simulink model "HDVPSG_DelayComp_NewRef_RealDrop_case1"  (R2019b)
settings: Solver=FixedStepDiscrete  StartTime=0.0  StopTime=28  FixedStep=UT.Ts_Veh  RelTol=1e-3
PostLoadFcn:
  | if any(exist('dsrtsu_mdlpostloadfcn', 'file') ~= 0), dsrtsu_mdlpostloadfcn('Execute', bdroot); end
InitFcn:
  | , if any(exist('dsmpb_private', 'file') ~= 0), dsmpb_private('dsmpb_mdlclblib', 'Init', bdroot); end,
values from neighbouring files (symbols this model uses):
  BETA_HDV_Leader = 50    [HDVPSG_DelayComp_NewRef_RealDrop_script_case1.m]
  BETA_PSG_Follower = 150    [HDVPSG_DelayComp_NewRef_RealDrop_script_case1.m]
  CtrlZone_Length = 250    [HDVPSG_DelayComp_NewRef_RealDrop_script_case1.m]
  DELTA_D_MIN = 5    [HDVPSG_DelayComp_NewRef_RealDrop_script_case1.m]
  DELTA_DR_MG_TCC = 15    [HDVPSG_DelayComp_NewRef_RealDrop_script_case1.m]
  HDV_AMAX = 1.3    [HDVPSG_DelayComp_NewRef_RealDrop_script_case1.m]
  HDV_AMIN = -2.5    [HDVPSG_DelayComp_NewRef_RealDrop_script_case1.m]
  HDV_first_v0 = 13    [HDVPSG_DelayComp_NewRef_RealDrop_script_case1.m]
  HDV_HighMu_D = 9    [HDVPSG_DelayComp_NewRef_RealDrop_script_case1.m]
  HDV_HighMu_I = 27    [HDVPSG_DelayComp_NewRef_RealDrop_script_case1.m]
  HDV_HighMu_P = 27    [HDVPSG_DelayComp_NewRef_RealDrop_script_case1.m]
  HDV_HighMu_TRFC = 0.7    [HDVPSG_DelayComp_NewRef_RealDrop_script_case1.m]
  HDV_last_v0 = 13    [HDVPSG_DelayComp_NewRef_RealDrop_script_case1.m]
  HDV_LowMu_D = 6    [HDVPSG_DelayComp_NewRef_RealDrop_script_case1.m]
  HDV_LowMu_I = 8    [HDVPSG_DelayComp_NewRef_RealDrop_script_case1.m]
  HDV_LowMu_P = 12    [HDVPSG_DelayComp_NewRef_RealDrop_script_case1.m]
  HDV_LowMu_TRFC = 0.6    [HDVPSG_DelayComp_NewRef_RealDrop_script_case1.m]
  Np_MPC = 20    [HDVPSG_DelayComp_NewRef_RealDrop_script_case1.m]
  PSG_AMAX = 3.2    [HDVPSG_DelayComp_NewRef_RealDrop_script_case1.m]
  PSG_AMIN = -6    [HDVPSG_DelayComp_NewRef_RealDrop_script_case1.m]
  PSG_end_v0 = 13    [HDVPSG_DelayComp_NewRef_RealDrop_script_case1.m]
  PSG_first_v0 = 13    [HDVPSG_DelayComp_NewRef_RealDrop_script_case1.m]
  PSG_HighMu_D = 15    [HDVPSG_DelayComp_NewRef_RealDrop_script_case1.m]
  PSG_HighMu_I = 125    [HDVPSG_DelayComp_NewRef_RealDrop_script_case1.m]
  PSG_HighMu_P = 75    [HDVPSG_DelayComp_NewRef_RealDrop_script_case1.m]
  PSG_HighMu_TRFC = 0.8    [HDVPSG_DelayComp_NewRef_RealDrop_script_case1.m]
  PSG_LowMu_D = 12    [HDVPSG_DelayComp_NewRef_RealDrop_script_case1.m]
  PSG_LowMu_I = 64    [HDVPSG_DelayComp_NewRef_RealDrop_script_case1.m]
  PSG_LowMu_P = 48    [HDVPSG_DelayComp_NewRef_RealDrop_script_case1.m]
  PSG_LowMu_TRFC = 0.7    [HDVPSG_DelayComp_NewRef_RealDrop_script_case1.m]
  PSG_middle_v0 = 13    [HDVPSG_DelayComp_NewRef_RealDrop_script_case1.m]
  Q_Leader = 1    [HDVPSG_DelayComp_NewRef_RealDrop_script_case1.m]
  Qd_dot_PSG_Follower = 2    [HDVPSG_DelayComp_NewRef_RealDrop_script_case1.m]
  Qd_PSG_Follower = 10    [HDVPSG_DelayComp_NewRef_RealDrop_script_case1.m]
  R_Leader = 20    [HDVPSG_DelayComp_NewRef_RealDrop_script_case1.m]
  R_PSG_Follower = 1    [HDVPSG_DelayComp_NewRef_RealDrop_script_case1.m]
  Recved_40_1 = Recved_Flag_Combined(47740,:)    [HDVPSG_DelayComp_NewRef_RealDrop_script_case1.m]
  Recved_40_2 = Recved_Flag_Combined(47780,:)    [HDVPSG_DelayComp_NewRef_RealDrop_script_case1.m]
  Recved_40_3 = Recved_Flag_Combined(49536,:)    [HDVPSG_DelayComp_NewRef_RealDrop_script_case1.m]
  Recved_40_4 = Recved_Flag_Combined(118106,:)    [HDVPSG_DelayComp_NewRef_RealDrop_script_case1.m]
  Rho_deltad_PSG_Follower = 1e3    (= 1000)    [HDVPSG_DelayComp_NewRef_RealDrop_script_case1.m]
  Rho_v_PSG_Follower = 1e3    (= 1000)    [HDVPSG_DelayComp_NewRef_RealDrop_script_case1.m]
  T_ADE = 0.01    [HDVPSG_DelayComp_NewRef_RealDrop_script_case1.m]
  V_MAX = 40    [HDVPSG_DelayComp_NewRef_RealDrop_script_case1.m]
  V_MIN = 0    [HDVPSG_DelayComp_NewRef_RealDrop_script_case1.m]
  VR_MG_TCC = 15    [HDVPSG_DelayComp_NewRef_RealDrop_script_case1.m]
undefined symbols (not defined in the file or in its folder): DiscIntNeverNeededParam, UT
libraries: simulink x46
(part 15 of 16)

== matlab function HDVPSG_DelayComp_NewRef_RealDrop_case1/ARE_First_Order_Derivative_[1,0,0]9/MATLAB Function ==
  data: U input; Dot_U output; Ts input; u_init input
function Dot_U = buffer(U, Ts, u_init)
    N = 12;
    %Ts = 0.01;
    persistent y;
    if isempty(y)
        y=u_init*ones(N+1,1);%m/s
    end

    y = [U;y(1:end-1)];
    T = Ts*N;
    P = zeros(1,N+1);
    P_alpha = P;
    for k = 1:N+1
        tao_k = (k-1)*Ts;
        P(k) = T-2*tao_k;
        if((k==1)||(k==N+1))
            P_alpha(k) = P(k)*Ts/2;
        else
            P_alpha(k) = P(k)*Ts;
        end
    end
    
    Dot_U = P_alpha*y*6/(T^3);

end

== matlab function HDVPSG_DelayComp_NewRef_RealDrop_case1/PSG2_control_withPDR_compen/Sys3 ==
  data: Ts input; A output; B output; dk output; beta input; delta_d_ddot_hat input
function [A, B, dk] = Sys(Ts, beta, delta_d_ddot_hat)
    A = [1  Ts;
         0  1];
    
    B =  [0; -beta*Ts];
    
    dk = [0; delta_d_ddot_hat*Ts];
end

== matlab function HDVPSG_DelayComp_NewRef_RealDrop_case1/HDV2_control_withPDR_compen/SELF_Optimal_Control_Reference ==
  data: opt_spd output; L_ctz input; opt_pos output; v_ini input; a_ini input; T_all_to_MP input; v_mp input; t_aft_trigger input; opt_acc output; opt_pos_vec output; opt_spd_vec output; alpha output; beta output; c_1 output; c_2 output; c_3 output; c_4 output
function [opt_spd, opt_pos, opt_acc, opt_pos_vec, opt_spd_vec, alpha, beta, c_1, c_2, c_3, c_4] = Opt_Ref(L_ctz, v_ini, a_ini, T_all_to_MP, v_mp, t_aft_trigger)
Np          = 20;
opt_pos_vec = zeros(1, Np+1);
opt_spd_vec = zeros(1, Np+1);
%opt_acc_vec = zeros(1, Np+1);

Ts    = 0.01;
L_ctz = -L_ctz;

alpha = -(12*v_mp - 12*v_ini - 12*L_ctz - 6*T_all_to_MP*a_ini - 12*T_all_to_MP*v_mp + 6*T_all_to_MP*L_ctz + 2*T_all_to_MP^2*a_ini + 2*T_all_to_MP^2*v_ini + 4*T_all_to_MP^2*v_mp + 12*v_ini*exp(-T_all_to_MP) - 12*v_mp*exp(-T_all_to_MP) + 12*L_ctz*exp(-T_all_to_MP) + 6*T_all_to_MP*a_ini*exp(-T_all_to_MP) + 12*T_all_to_MP*v_ini*exp(-T_all_to_MP) + 6*T_all_to_MP*L_ctz*exp(-T_all_to_MP) + 4*T_all_to_MP^2*a_ini*exp(-T_all_to_MP) + T_all_to_MP^3*a_ini*exp(-T_all_to_MP) + 4*T_all_to_MP^2*v_ini*exp(-T_all_to_MP) + 2*T_all_to_MP^2*v_mp*exp(-T_all_to_MP))/(24*exp(-T_all_to_MP) + 24*exp(T_all_to_MP) + 8*T_all_to_MP^2*exp(-T_all_to_MP) + T_all_to_MP^3*exp(-T_all_to_MP) - 24*T_all_to_MP*exp(T_all_to_MP) + 8*T_all_to_MP^2 + 24*T_all_to_MP*exp(-T_all_to_MP) + 8*T_all_to_MP^2*exp(T_all_to_MP) - T_all_to_MP^3*exp(T_all_to_MP) - 48);

beta  = -(12*v_mp - 12*v_ini + 12*L_ctz - 6*T_all_to_MP*a_ini + 12*T_all_to_MP*v_mp + 6*T_all_to_MP*L_ctz - 2*T_all_to_MP^2*a_ini + 2*T_all_to_MP^2*v_ini + 4*T_all_to_MP^2*v_mp + 12*v_ini*exp(T_all_to_MP) - 12*v_mp*exp(T_all_to_MP) - 12*L_ctz*exp(T_all_to_MP) - 4*T_all_to_MP^2*a_ini*exp(T_all_to_MP) + T_all_to_MP^3*a_ini*exp(T_all_to_MP) + 4*T_all_to_MP^2*v_ini*exp(T_all_to_MP) + 2*T_all_to_MP^2*v_mp*exp(T_all_to_MP) + 6*T_all_to_MP*a_ini*exp(T_all_to_MP) - 12*T_all_to_MP*v_ini*exp(T_all_to_MP) + 6*T_all_to_MP*L_ctz*exp(T_all_to_MP))/(24*exp(-T_all_to_MP) + 24*exp(T_all_to_MP) + 8*T_all_to_MP^2*exp(-T_all_to_MP) + T_all_to_MP^3*exp(-T_all_to_MP) - 24*T_all_to_MP*exp(T_all_to_MP) + 8*T_all_to_MP^2 + 24*T_all_to_MP*exp(-T_all_to_MP) + 8*T_all_to_MP^2*exp(T_all_to_MP) - T_all_to_MP^3*exp(T_all_to_MP) - 48);

  c_1 = -(6*(8*L_ctz - 8*a_ini + 4*T_all_to_MP*v_ini + 4*T_all_to_MP*v_mp + 2*T_all_to_MP^2*a_ini + 4*a_ini*exp(T_all_to_MP) - 4*L_ctz*exp(T_all_to_MP) + 4*a_ini*exp(-T_all_to_MP) - 4*L_ctz*exp(-T_all_to_MP) + 4*T_all_to_MP*a_ini*exp(-T_all_to_MP) + T_all_to_MP^2*a_ini*exp(T_all_to_MP) - 2*T_all_to_MP*v_ini*exp(-T_all_to_MP) + T_all_to_MP^2*v_ini*exp(T_all_to_MP) - 2*T_all_to_MP*v_mp*exp(-T_all_to_MP) + T_all_to_MP^2*v_mp*exp(T_all_to_MP) - 2*T_all_to_MP*L_ctz*exp(-T_all_to_MP) + T_all_to_MP^2*a_ini*exp(-T_all_to_MP) - T_all_to_MP^2*v_ini*exp(-T_all_to_MP) - T_all_to_MP^2*v_mp*exp(-T_all_to_MP) - 4*T_all_to_MP*a_ini*exp(T_all_to_MP) - 2*T_all_to_MP*v_ini*exp(T_all_to_MP) - 2*T_all_to_MP*v_mp*exp(T_all_to_MP) + 2*T_all_to_MP*L_ctz*exp(T_all_to_MP)))/(T_all_to_MP*(24*exp(-T_all_to_MP) + 24*exp(T_all_to_MP) + 8*T_all_to_MP^2*exp(-T_all_to_MP) + T_all_to_MP^3*exp(-T_all_to_MP) - 24*T_all_to_MP*exp(T_all_to_MP) + 8*T_all_to_MP^2 + 24*T_all_to_MP*exp(-T_all_to_MP) + 8*T_all_to_MP^2*exp(T_all_to_MP) - T_all_to_MP^3*exp(T_all_to_MP) - 48)); 
  
  c_2 = (2*(12*L_ctz - 24*a_ini + 12*T_all_to_MP*v_mp + 2*T_all_to_MP^2*a_ini + 12*a_ini*exp(T_all_to_MP) + 6*v_ini*exp(T_all_to_MP) - 6*v_mp*exp(T_all_to_MP) - 6*L_ctz*exp(T_all_to_MP) + 12*a_ini*exp(-T_all_to_MP) - 6*v_ini*exp(-T_all_to_MP) + 6*v_mp*exp(-T_all_to_MP) - 6*L_ctz*exp(-T_all_to_MP) + 9*T_all_to_MP*a_ini*exp(-T_all_to_MP) + 2*T_all_to_MP^2*a_ini*exp(T_all_to_MP) - 6*T_all_to_MP*v_ini*exp(-T_all_to_MP) + 2*T_all_to_MP^2*v_ini*exp(T_all_to_MP) + T_all_to_MP^2*v_mp*exp(T_all_to_MP) - 3*T_all_to_MP*L_ctz*exp(-T_all_to_MP) + 2*T_all_to_MP^2*a_ini*exp(-T_all_to_MP) - 2*T_all_to_MP^2*v_ini*exp(-T_all_to_MP) - T_all_to_MP^2*v_mp*exp(-T_all_to_MP) - 9*T_all_to_MP*a_ini*exp(T_all_to_MP) - 6*T_all_to_MP*v_ini*exp(T_all_to_MP) + 3*T_all_to_MP*L_ctz*exp(T_all_to_MP)))/(24*exp(-T_all_to_MP) + 24*exp(T_all_to_MP) + 8*T_all_to_MP^2*exp(-T_all_to_MP) + T_all_to_MP^3*exp(-T_all_to_MP) - 24*T_all_to_MP*exp(T_all_to_MP) + 8*T_all_to_MP^2 + 24*T_all_to_MP*exp(-T_all_to_MP) + 8*T_all_to_MP^2*exp(T_all_to_MP) - T_all_to_MP^3*exp(T_all_to_MP) - 48); 
  
  c_3 = -(24*v_ini + 24*v_mp - 12*T_all_to_MP*a_ini + 12*T_all_to_MP*L_ctz - 4*T_all_to_MP^2*v_ini + 8*T_all_to_MP^2*v_mp - 12*v_ini*exp(T_all_to_MP) - 12*v_mp*exp(T_all_to_MP) - 12*L_ctz*exp(T_all_to_MP) - 12*v_ini*exp(-T_all_to_MP) - 12*v_mp*exp(-T_all_to_MP) + 12*L_ctz*exp(-T_all_to_MP) + 6*T_all_to_MP*a_ini*exp(-T_all_to_MP) - 4*T_all_to_MP^2*a_ini*exp(T_all_to_MP) + T_all_to_MP^3*a_ini*exp(T_all_to_MP) - 12*T_all_to_MP*v_ini*exp(-T_all_to_MP) - 4*T_all_to_MP^2*v_ini*exp(T_all_to_MP) + T_all_to_MP^3*v_ini*exp(T_all_to_MP) + 2*T_all_to_MP^2*v_mp*exp(T_all_to_MP) + 6*T_all_to_MP*L_ctz*exp(-T_all_to_MP) + 4*T_all_to_MP^2*a_ini*exp(-T_all_to_MP) + T_all_to_MP^3*a_ini*exp(-T_all_to_MP) - 4*T_all_to_MP^2*v_ini*exp(-T_all_to_MP) - T_all_to_MP^3*v_ini*exp(-T_all_to_MP) + 2*T_all_to_MP^2*v_mp*exp(-T_all_to_MP) + 6*T_all_to_MP*a_ini*exp(T_all_to_MP) + 12*T_all_to_MP*v_ini*exp(T_all_to_MP) + 6*T_all_to_MP*L_ctz*exp(T_all_to_MP))/(24*exp(-T_all_to_MP) + 24*exp(T_all_to_MP) + 8*T_all_to_MP^2*exp(-T_all_to_MP) + T_all_to_MP^3*exp(-T_all_to_MP) - 24*T_all_to_MP*exp(T_all_to_MP) + 8*T_all_to_MP^2 + 24*T_all_to_MP*exp(-T_all_to_MP) + 8*T_all_to_MP^2*exp(T_all_to_MP) - T_all_to_MP^3*exp(T_all_to_MP) - 48); 
  
  c_4 = -(24*L_ctz - 24*T_all_to_MP*v_mp + 4*T_all_to_MP^2*a_ini - 8*T_all_to_MP^2*L_ctz - 12*v_ini*exp(T_all_to_MP) + 12*v_mp*exp(T_all_to_MP) - 12*L_ctz*exp(T_all_to_MP) + 12*v_ini*exp(-T_all_to_MP) - 12*v_mp*exp(-T_all_to_MP) - 12*L_ctz*exp(-T_all_to_MP) + 6*T_all_to_MP*a_ini*exp(-T_all_to_MP) + 4*T_all_to_MP^2*a_ini*exp(T_all_to_MP) - T_all_to_MP^3*a_ini*exp(T_all_to_MP) + 12*T_all_to_MP*v_ini*exp(-T_all_to_MP) - 4*T_all_to_MP^2*v_ini*exp(T_all_to_MP) - 2*T_all_to_MP^2*v_mp*exp(T_all_to_MP) - 18*T_all_to_MP*L_ctz*exp(-T_all_to_MP) - 8*T_all_to_MP^2*L_ctz*exp(T_all_to_MP) + T_all_to_MP^3*L_ctz*exp(T_all_to_MP) + 4*T_all_to_MP^2*a_ini*exp(-T_all_to_MP) + T_all_to_MP^3*a_ini*exp(-T_all_to_MP) + 4*T_all_to_MP^2*v_ini*exp(-T_all_to_MP) + 2*T_all_to_MP^2*v_mp*exp(-T_all_to_MP) - 8*T_all_to_MP^2*L_ctz*exp(-T_all_to_MP) - T_all_to_MP^3*L_ctz*exp(-T_all_to_MP) - 6*T_all_to_MP*a_ini*exp(T_all_to_MP) + 12*T_all_to_MP*v_ini*exp(T_all_to_MP) + 18*T_all_to_MP*L_ctz*exp(T_all_to_MP))/(24*exp(-T_all_to_MP) + 24*exp(T_all_to_MP) + 8*T_all_to_MP^2*exp(-T_all_to_MP) + T_all_to_MP^3*exp(-T_all_to_MP) - 24*T_all_to_MP*exp(T_all_to_MP) + 8*T_all_to_MP^2 + 24*T_all_to_MP*exp(-T_all_to_MP) + 8*T_all_to_MP^2*exp(T_all_to_MP) - T_all_to_MP^3*exp(T_all_to_MP) - 48);
  
 % t = min(t, T_rest_to_MP);
  t_vec = t_aft_trigger + (1:(Np+1))*Ts;
 
 if t_aft_trigger <= T_all_to_MP
     opt_pos = -alpha.*exp(t_aft_trigger) + beta.*exp(-t_aft_trigger) + 1/6.*c_1.*t_aft_trigger.^3 + c_2./2.*t_aft_trigger.^2 + c_3.*t_aft_trigger + c_4;
     opt_spd = -alpha.*exp(t_aft_trigger) - beta.*exp(-t_aft_trigger) + 1/2.*c_1.*t_aft_trigger.^2 + c_2.*t_aft_trigger + c_3;
     opt_acc = -alpha.*exp(t_aft_trigger) + beta.*exp(-t_aft_trigger) + c_1.*t_aft_trigger + c_2;
 else
     opt_pos = v_mp*(t_aft_trigger-T_all_to_MP);
     opt_spd = v_mp;
     opt_acc = 0;
 end
 
for i = 1:Np+1
    if t_vec(i)<=T_all_to_MP
        opt_pos_vec(i) = -alpha.*exp(t_vec(i)) + beta.*exp(-t_vec(i)) + 1/6.*c_1.*t_vec(i).^3 + c_2./2.*t_vec(i).^2 + c_3.*t_vec(i) + c_4;
        opt_spd_vec(i) = -alpha.*exp(t_vec(i)) - beta.*exp(-t_vec(i)) + 1/2.*c_1.*t_vec(i).^2 + c_2.*t_vec(i)       + c_3;
      %  opt_acc_vec(i) = -alpha.*exp(t_vec(i)) + beta.*exp(-t_vec(i)) + c_1.*t_vec(i) + c_2;
    else
        opt_pos_vec(i) = v_mp*(t_vec(i)-T_all_to_MP); 
        opt_spd_vec(i) = v_mp;
     %   opt_acc_vec(i) = 0; 
    end
end
 
end

== matlab function HDVPSG_DelayComp_NewRef_RealDrop_case1/leader_ulmpc_spd_ctrl/Sys_Leader ==
  data: Ts input; A output; B output; dk output; beta input; v_dot_hat input
function [A,B,dk] = f(Ts, beta, v_dot_hat)
    A  = 1;
    B  = beta*Ts;
    dk = v_dot_hat*Ts;
end

== matlab function HDVPSG_DelayComp_NewRef_RealDrop_case1/PSG3_control_withPDR_compen/MATLAB Function2 ==
  data: Recv input; Lost_Step output
function Lost_Step = fcn(Recv)
  persistent NUM;
  if isempty(NUM)
      NUM =0;
  end
      
  if Recv == 0
      NUM = NUM +1;
  else
      NUM = 0;
  end
  Lost_Step = NUM;
end

== matlab function HDVPSG_DelayComp_NewRef_RealDrop_case1/ARE_First_Order_Derivative_[1,0,0]10/MATLAB Function ==
  data: U input; Dot_U output; Ts input; u_init input
function Dot_U = buffer(U, Ts, u_init)
    N = 12;
    %Ts = 0.01;
    persistent y;
    if isempty(y)
        y=u_init*ones(N+1,1);%m/s
    end

    y = [U;y(1:end-1)];
    T = Ts*N;
    P = zeros(1,N+1);
    P_alpha = P;
    for k = 1:N+1
        tao_k = (k-1)*Ts;
        P(k) = T-2*tao_k;
        if((k==1)||(k==N+1))
            P_alpha(k) = P(k)*Ts/2;
        else
            P_alpha(k) = P(k)*Ts;
        end
    end
    
    Dot_U = P_alpha*y*6/(T^3);

end

== matlab function HDVPSG_DelayComp_NewRef_RealDrop_case1/ARE_First_Order_Derivative_[1,0,0]7/MATLAB Function ==
  data: U input; Dot_U output; Ts input; u_init input
function Dot_U = buffer(U, Ts, u_init)
    N = 12;
    %Ts = 0.01;
    persistent y;
    if isempty(y)
        y=u_init*ones(N+1,1);%m/s
    end

    y = [U;y(1:end-1)];
    T = Ts*N;
    P = zeros(1,N+1);
    P_alpha = P;
    for k = 1:N+1
        tao_k = (k-1)*Ts;
        P(k) = T-2*tao_k;
        if((k==1)||(k==N+1))
            P_alpha(k) = P(k)*Ts/2;
        else
            P_alpha(k) = P(k)*Ts;
        end
    end
    
    Dot_U = P_alpha*y*6/(T^3);

end

== matlab function HDVPSG_DelayComp_NewRef_RealDrop_case1/PSG3_control_withPDR_compen/PRE_OPT_Pos ==
  data: alpha_pre input; opt_pos_pre output; opt_spd_pre output; beta_pre input; c_1_pre input; c_2_pre input; c_3_pre input; c_4_pre input; v_mp input; T_all_to_MP_pre input; t_aft_trigger_pre input; opt_pos_pre_vec output; opt_spd_pre_vec output
function [opt_pos_pre, opt_spd_pre, opt_pos_pre_vec, opt_spd_pre_vec] = Opt_Pos_Ref_Pre(alpha_pre, beta_pre, c_1_pre, c_2_pre, c_3_pre, c_4_pre, v_mp, T_all_to_MP_pre, t_aft_trigger_pre)
Np              = 20;
opt_pos_pre_vec = zeros(1, Np+1);
opt_spd_pre_vec = zeros(1, Np+1);
%opt_acc_vec = zeros(1, Np+1);

Ts    = 0.01;
 % t = min(t, T_rest_to_MP);
  t_vec = t_aft_trigger_pre + (1:(Np+1))*Ts;
 
 if t_aft_trigger_pre <= T_all_to_MP_pre
     opt_pos_pre = -alpha_pre.*exp(t_aft_trigger_pre) + beta_pre.*exp(-t_aft_trigger_pre) + 1/6.*c_1_pre.*t_aft_trigger_pre.^3 + c_2_pre./2.*t_aft_trigger_pre.^2 + c_3_pre.*t_aft_trigger_pre + c_4_pre;
     opt_spd_pre = -alpha_pre.*exp(t_aft_trigger_pre) - beta_pre.*exp(-t_aft_trigger_pre) + 1/2.*c_1_pre.*t_aft_trigger_pre.^2 + c_2_pre.*t_aft_trigger_pre + c_3_pre;
 else
     opt_pos_pre = v_mp*(t_aft_trigger_pre-T_all_to_MP_pre);
     opt_spd_pre = v_mp;
 end
 
for i = 1:Np+1
    if t_vec(i)<=T_all_to_MP_pre
        opt_pos_pre_vec(i) = -alpha_pre.*exp(t_vec(i)) + beta_pre.*exp(-t_vec(i)) + 1/6.*c_1_pre.*t_vec(i).^3 + c_2_pre./2.*t_vec(i).^2 + c_3_pre.*t_vec(i) + c_4_pre;
        opt_spd_pre_vec(i) = -alpha_pre.*exp(t_vec(i)) - beta_pre.*exp(-t_vec(i)) + 1/2.*c_1_pre.*t_vec(i).^2 + c_2_pre.*t_vec(i)       + c_3_pre;
      %  opt_acc_vec(i) = -alpha.*exp(t_vec(i)) + beta.*exp(-t_vec(i)) + c_1.*t_vec(i) + c_2;
    else
        opt_pos_pre_vec(i) = v_mp*(t_vec(i)-T_all_to_MP_pre); 
        opt_spd_pre_vec(i) = v_mp;
     %   opt_acc_vec(i) = 0; 
    end
end
 
end

== matlab function HDVPSG_DelayComp_NewRef_RealDrop_case1/HDV2_control_withPDR_compen/MATLAB Function ==
  data: REALWORLD_DIST output; X_Ego input; Rho_delta_d_adpt output; Y_Ego input; X_Front input; Y_Front input; DELTA_D_MIN input; Rho_delta_dMAX input
function [REALWORLD_DIST, Rho_delta_d_adpt] = Adaptive_Rho_delta_d(X_Ego, Y_Ego, X_Front, Y_Front, DELTA_D_MIN, Rho_delta_dMAX)
    REALWORLD_DIST = sqrt((X_Ego - X_Front)^2 + (Y_Ego - Y_Front)^2); % The virtual leading car may be in another lane: So far away from the ego_car

    if REALWORLD_DIST>2*DELTA_D_MIN  %  This is determined by the road geometry
        Rho_delta_d_adpt = 0; % Disable 
    elseif REALWORLD_DIST>DELTA_D_MIN
        Rho_delta_d_adpt = -Rho_delta_dMAX/DELTA_D_MIN*REALWORLD_DIST + 2*Rho_delta_dMAX;   % linear adaptive gain
    else
        Rho_delta_d_adpt = Rho_delta_dMAX;
    end
    
end

== matlab function HDVPSG_DelayComp_NewRef_RealDrop_case1/PSG3_control_withPDR_compen/SELF_Optimal_Control_Reference ==
  data: opt_spd output; L_ctz input; opt_pos output; v_ini input; a_ini input; T_all_to_MP input; v_mp input; t_aft_trigger input; opt_acc output; opt_pos_vec output; opt_spd_vec output; alpha output; beta output; c_1 output; c_2 output; c_3 output; c_4 output
function [opt_spd, opt_pos, opt_acc, opt_pos_vec, opt_spd_vec, alpha, beta, c_1, c_2, c_3, c_4] = Opt_Ref(L_ctz, v_ini, a_ini, T_all_to_MP, v_mp, t_aft_trigger)
Np          = 20;
opt_pos_vec = zeros(1, Np+1);
opt_spd_vec = zeros(1, Np+1);
%opt_acc_vec = zeros(1, Np+1);

Ts    = 0.01;
L_ctz = -L_ctz;

alpha = -(12*v_mp - 12*v_ini - 12*L_ctz - 6*T_all_to_MP*a_ini - 12*T_all_to_MP*v_mp + 6*T_all_to_MP*L_ctz + 2*T_all_to_MP^2*a_ini + 2*T_all_to_MP^2*v_ini + 4*T_all_to_MP^2*v_mp + 12*v_ini*exp(-T_all_to_MP) - 12*v_mp*exp(-T_all_to_MP) + 12*L_ctz*exp(-T_all_to_MP) + 6*T_all_to_MP*a_ini*exp(-T_all_to_MP) + 12*T_all_to_MP*v_ini*exp(-T_all_to_MP) + 6*T_all_to_MP*L_ctz*exp(-T_all_to_MP) + 4*T_all_to_MP^2*a_ini*exp(-T_all_to_MP) + T_all_to_MP^3*a_ini*exp(-T_all_to_MP) + 4*T_all_to_MP^2*v_ini*exp(-T_all_to_MP) + 2*T_all_to_MP^2*v_mp*exp(-T_all_to_MP))/(24*exp(-T_all_to_MP) + 24*exp(T_all_to_MP) + 8*T_all_to_MP^2*exp(-T_all_to_MP) + T_all_to_MP^3*exp(-T_all_to_MP) - 24*T_all_to_MP*exp(T_all_to_MP) + 8*T_all_to_MP^2 + 24*T_all_to_MP*exp(-T_all_to_MP) + 8*T_all_to_MP^2*exp(T_all_to_MP) - T_all_to_MP^3*exp(T_all_to_MP) - 48);

beta  = -(12*v_mp - 12*v_ini + 12*L_ctz - 6*T_all_to_MP*a_ini + 12*T_all_to_MP*v_mp + 6*T_all_to_MP*L_ctz - 2*T_all_to_MP^2*a_ini + 2*T_all_to_MP^2*v_ini + 4*T_all_to_MP^2*v_mp + 12*v_ini*exp(T_all_to_MP) - 12*v_mp*exp(T_all_to_MP) - 12*L_ctz*exp(T_all_to_MP) - 4*T_all_to_MP^2*a_ini*exp(T_all_to_MP) + T_all_to_MP^3*a_ini*exp(T_all_to_MP) + 4*T_all_to_MP^2*v_ini*exp(T_all_to_MP) + 2*T_all_to_MP^2*v_mp*exp(T_all_to_MP) + 6*T_all_to_MP*a_ini*exp(T_all_to_MP) - 12*T_all_to_MP*v_ini*exp(T_all_to_MP) + 6*T_all_to_MP*L_ctz*exp(T_all_to_MP))/(24*exp(-T_all_to_MP) + 24*exp(T_all_to_MP) + 8*T_all_to_MP^2*exp(-T_all_to_MP) + T_all_to_MP^3*exp(-T_all_to_MP) - 24*T_all_to_MP*exp(T_all_to_MP) + 8*T_all_to_MP^2 + 24*T_all_to_MP*exp(-T_all_to_MP) + 8*T_all_to_MP^2*exp(T_all_to_MP) - T_all_to_MP^3*exp(T_all_to_MP) - 48);

  c_1 = -(6*(8*L_ctz - 8*a_ini + 4*T_all_to_MP*v_ini + 4*T_all_to_MP*v_mp + 2*T_all_to_MP^2*a_ini + 4*a_ini*exp(T_all_to_MP) - 4*L_ctz*exp(T_all_to_MP) + 4*a_ini*exp(-T_all_to_MP) - 4*L_ctz*exp(-T_all_to_MP) + 4*T_all_to_MP*a_ini*exp(-T_all_to_MP) + T_all_to_MP^2*a_ini*exp(T_all_to_MP) - 2*T_all_to_MP*v_ini*exp(-T_all_to_MP) + T_all_to_MP^2*v_ini*exp(T_all_to_MP) - 2*T_all_to_MP*v_mp*exp(-T_all_to_MP) + T_all_to_MP^2*v_mp*exp(T_all_to_MP) - 2*T_all_to_MP*L_ctz*exp(-T_all_to_MP) + T_all_to_MP^2*a_ini*exp(-T_all_to_MP) - T_all_to_MP^2*v_ini*exp(-T_all_to_MP) - T_all_to_MP^2*v_mp*exp(-T_all_to_MP) - 4*T_all_to_MP*a_ini*exp(T_all_to_MP) - 2*T_all_to_MP*v_ini*exp(T_all_to_MP) - 2*T_all_to_MP*v_mp*exp(T_all_to_MP) + 2*T_all_to_MP*L_ctz*exp(T_all_to_MP)))/(T_all_to_MP*(24*exp(-T_all_to_MP) + 24*exp(T_all_to_MP) + 8*T_all_to_MP^2*exp(-T_all_to_MP) + T_all_to_MP^3*exp(-T_all_to_MP) - 24*T_all_to_MP*exp(T_all_to_MP) + 8*T_all_to_MP^2 + 24*T_all_to_MP*exp(-T_all_to_MP) + 8*T_all_to_MP^2*exp(T_all_to_MP) - T_all_to_MP^3*exp(T_all_to_MP) - 48)); 
  
  c_2 = (2*(12*L_ctz - 24*a_ini + 12*T_all_to_MP*v_mp + 2*T_all_to_MP^2*a_ini + 12*a_ini*exp(T_all_to_MP) + 6*v_ini*exp(T_all_to_MP) - 6*v_mp*exp(T_all_to_MP) - 6*L_ctz*exp(T_all_to_MP) + 12*a_ini*exp(-T_all_to_MP) - 6*v_ini*exp(-T_all_to_MP) + 6*v_mp*exp(-T_all_to_MP) - 6*L_ctz*exp(-T_all_to_MP) + 9*T_all_to_MP*a_ini*exp(-T_all_to_MP) + 2*T_all_to_MP^2*a_ini*exp(T_all_to_MP) - 6*T_all_to_MP*v_ini*exp(-T_all_to_MP) + 2*T_all_to_MP^2*v_ini*exp(T_all_to_MP) + T_all_to_MP^2*v_mp*exp(T_all_to_MP) - 3*T_all_to_MP*L_ctz*exp(-T_all_to_MP) + 2*T_all_to_MP^2*a_ini*exp(-T_all_to_MP) - 2*T_all_to_MP^2*v_ini*exp(-T_all_to_MP) - T_all_to_MP^2*v_mp*exp(-T_all_to_MP) - 9*T_all_to_MP*a_ini*exp(T_all_to_MP) - 6*T_all_to_MP*v_ini*exp(T_all_to_MP) + 3*T_all_to_MP*L_ctz*exp(T_all_to_MP)))/(24*exp(-T_all_to_MP) + 24*exp(T_all_to_MP) + 8*T_all_to_MP^2*exp(-T_all_to_MP) + T_all_to_MP^3*exp(-T_all_to_MP) - 24*T_all_to_MP*exp(T_all_to_MP) + 8*T_all_to_MP^2 + 24*T_all_to_MP*exp(-T_all_to_MP) + 8*T_all_to_MP^2*exp(T_all_to_MP) - T_all_to_MP^3*exp(T_all_to_MP) - 48); 
  
  c_3 = -(24*v_ini + 24*v_mp - 12*T_all_to_MP*a_ini + 12*T_all_to_MP*L_ctz - 4*T_all_to_MP^2*v_ini + 8*T_all_to_MP^2*v_mp - 12*v_ini*exp(T_all_to_MP) - 12*v_mp*exp(T_all_to_MP) - 12*L_ctz*exp(T_all_to_MP) - 12*v_ini*exp(-T_all_to_MP) - 12*v_mp*exp(-T_all_to_MP) + 12*L_ctz*exp(-T_all_to_MP) + 6*T_all_to_MP*a_ini*exp(-T_all_to_MP) - 4*T_all_to_MP^2*a_ini*exp(T_all_to_MP) + T_all_to_MP^3*a_ini*exp(T_all_to_MP) - 12*T_all_to_MP*v_ini*exp(-T_all_to_MP) - 4*T_all_to_MP^2*v_ini*exp(T_all_to_MP) + T_all_to_MP^3*v_ini*exp(T_all_to_MP) + 2*T_all_to_MP^2*v_mp*exp(T_all_to_MP) + 6*T_all_to_MP*L_ctz*exp(-T_all_to_MP) + 4*T_all_to_MP^2*a_ini*exp(-T_all_to_MP) + T_all_to_MP^3*a_ini*exp(-T_all_to_MP) - 4*T_all_to_MP^2*v_ini*exp(-T_all_to_MP) - T_all_to_MP^3*v_ini*exp(-T_all_to_MP) + 2*T_all_to_MP^2*v_mp*exp(-T_all_to_MP) + 6*T_all_to_MP*a_ini*exp(T_all_to_MP) + 12*T_all_to_MP*v_ini*exp(T_all_to_MP) + 6*T_all_to_MP*L_ctz*exp(T_all_to_MP))/(24*exp(-T_all_to_MP) + 24*exp(T_all_to_MP) + 8*T_all_to_MP^2*exp(-T_all_to_MP) + T_all_to_MP^3*exp(-T_all_to_MP) - 24*T_all_to_MP*exp(T_all_to_MP) + 8*T_all_to_MP^2 + 24*T_all_to_MP*exp(-T_all_to_MP) + 8*T_all_to_MP^2*exp(T_all_to_MP) - T_all_to_MP^3*exp(T_all_to_MP) - 48); 
  
  c_4 = -(24*L_ctz - 24*T_all_to_MP*v_mp + 4*T_all_to_MP^2*a_ini - 8*T_all_to_MP^2*L_ctz - 12*v_ini*exp(T_all_to_MP) + 12*v_mp*exp(T_all_to_MP) - 12*L_ctz*exp(T_all_to_MP) + 12*v_ini*exp(-T_all_to_MP) - 12*v_mp*exp(-T_all_to_MP) - 12*L_ctz*exp(-T_all_to_MP) + 6*T_all_to_MP*a_ini*exp(-T_all_to_MP) + 4*T_all_to_MP^2*a_ini*exp(T_all_to_MP) - T_all_to_MP^3*a_ini*exp(T_all_to_MP) + 12*T_all_to_MP*v_ini*exp(-T_all_to_MP) - 4*T_all_to_MP^2*v_ini*exp(T_all_to_MP) - 2*T_all_to_MP^2*v_mp*exp(T_all_to_MP) - 18*T_all_to_MP*L_ctz*exp(-T_all_to_MP) - 8*T_all_to_MP^2*L_ctz*exp(T_all_to_MP) + T_all_to_MP^3*L_ctz*exp(T_all_to_MP) + 4*T_all_to_MP^2*a_ini*exp(-T_all_to_MP) + T_all_to_MP^3*a_ini*exp(-T_all_to_MP) + 4*T_all_to_MP^2*v_ini*exp(-T_all_to_MP) + 2*T_all_to_MP^2*v_mp*exp(-T_all_to_MP) - 8*T_all_to_MP^2*L_ctz*exp(-T_all_to_MP) - T_all_to_MP^3*L_ctz*exp(-T_all_to_MP) - 6*T_all_to_MP*a_ini*exp(T_all_to_MP) + 12*T_all_to_MP*v_ini*exp(T_all_to_MP) + 18*T_all_to_MP*L_ctz*exp(T_all_to_MP))/(24*exp(-T_all_to_MP) + 24*exp(T_all_to_MP) + 8*T_all_to_MP^2*exp(-T_all_to_MP) + T_all_to_MP^3*exp(-T_all_to_MP) - 24*T_all_to_MP*exp(T_all_to_MP) + 8*T_all_to_MP^2 + 24*T_all_to_MP*exp(-T_all_to_MP) + 8*T_all_to_MP^2*exp(T_all_to_MP) - T_all_to_MP^3*exp(T_all_to_MP) - 48);
  
 % t = min(t, T_rest_to_MP);
  t_vec = t_aft_trigger + (1:(Np+1))*Ts;
 
 if t_aft_trigger <= T_all_to_MP
     opt_pos = -alpha.*exp(t_aft_trigger) + beta.*exp(-t_aft_trigger) + 1/6.*c_1.*t_aft_trigger.^3 + c_2./2.*t_aft_trigger.^2 + c_3.*t_aft_trigger + c_4;
     opt_spd = -alpha.*exp(t_aft_trigger) - beta.*exp(-t_aft_trigger) + 1/2.*c_1.*t_aft_trigger.^2 + c_2.*t_aft_trigger + c_3;
     opt_acc = -alpha.*exp(t_aft_trigger) + beta.*exp(-t_aft_trigger) + c_1.*t_aft_trigger + c_2;
 else
     opt_pos = v_mp*(t_aft_trigger-T_all_to_MP);
     opt_spd = v_mp;
     opt_acc = 0;
 end
 
for i = 1:Np+1
    if t_vec(i)<=T_all_to_MP
        opt_pos_vec(i) = -alpha.*exp(t_vec(i)) + beta.*exp(-t_vec(i)) + 1/6.*c_1.*t_vec(i).^3 + c_2./2.*t_vec(i).^2 + c_3.*t_vec(i) + c_4;
        opt_spd_vec(i) = -alpha.*exp(t_vec(i)) - beta.*exp(-t_vec(i)) + 1/2.*c_1.*t_vec(i).^2 + c_2.*t_vec(i)       + c_3;
      %  opt_acc_vec(i) = -alpha.*exp(t_vec(i)) + beta.*exp(-t_vec(i)) + c_1.*t_vec(i) + c_2;
    else
        opt_pos_vec(i) = v_mp*(t_vec(i)-T_all_to_MP); 
        opt_spd_vec(i) = v_mp;
     %   opt_acc_vec(i) = 0; 
    end
end
 
end

== matlab function HDVPSG_DelayComp_NewRef_RealDrop_case1/PSG3_control_withPDR_compen/States_update2 ==
  data: x0 output; delta_d input; delta_d_dot input
function x0 = Init(delta_d, delta_d_dot)
    x0 = [delta_d;
          delta_d_dot];
end

== matlab function HDVPSG_DelayComp_NewRef_RealDrop_case1/PSG3_control_withPDR_compen/Subsystem17/Poly_coefficient ==
  data: a_0 output; delta_d0 input; a_1 output; a_2 output; delta_dTCC input; delta_v0 input; Tend input; a_3 output
function [a_0, a_1, a_2, a_3] = poly_4_coefficient(delta_d0, delta_dTCC, delta_v0, Tend)
% With conditions:
% delta_d_0 given,            delta_v_0 given 
% delta_d_Tend = delta_d_TTC, delta_v_Tend = 0

% delta_dr(t) = a0 + a1*t + a2*t^2 + a3*t^3
    a_0 = delta_d0;
    a_1 = delta_v0;
    a_2 = -(3*delta_d0 - 3*delta_dTCC + 2*Tend*delta_v0)/Tend^2;
    a_3 = (2*delta_d0 - 2*delta_dTCC + Tend*delta_v0)/Tend^3;
end

== matlab function HDVPSG_DelayComp_NewRef_RealDrop_case1/PSG3_control_withPDR_compen/Subsystem18/Ref ==
  data: delta_dr output; a_0 input; delta_dr_dot output; a_1 input; a_2 input; a_3 input; t_sumo input
function [delta_dr, delta_dr_dot] = poly_4_reference(a_0, a_1, a_2, a_3, t_sumo)
    delta_dr     = a_0 + a_1*t_sumo + a_2*t_sumo^2 + a_3*t_sumo^3;
    delta_dr_dot =       a_1        + 2*a_2*t_sumo + 3*a_3*t_sumo^2;
end

== matlab function HDVPSG_DelayComp_NewRef_RealDrop_case1/PSG3_control_withPDR_compen/Subsystem18/Ref_Pre_Vec ==
  data: delta_dr_Pre_Vec output; a_0 input; delta_dr_dot_Pre_Vec output; a_1 input; a_2 input; a_3 input; t_sumo input
function [delta_dr_Pre_Vec, delta_dr_dot_Pre_Vec] = poly_4_reference(a_0, a_1, a_2, a_3, t_sumo)
    Ts = 0.01;
    Np = 20;
    
    t_Pre_Vec = t_sumo + (1:Np+1)*Ts;
    
    delta_dr_Pre_Vec     = a_0 + a_1*t_Pre_Vec + a_2*t_Pre_Vec.^2 + a_3*t_Pre_Vec.^3;
    delta_dr_dot_Pre_Vec =       a_1           + 2*a_2*t_Pre_Vec  + 3*a_3*t_Pre_Vec.^2;
end

== matlab function HDVPSG_DelayComp_NewRef_RealDrop_case1/PSG2_control_withPDR_compen/Subsystem2/MATLAB Function3 ==
  data: Lost_Step input; delta_d_pre_freeze_if_lost input; delta_d_measure input; delta_d_MPC output
function delta_d_MPC  = fcn(Lost_Step, delta_d_pre_freeze_if_lost, delta_d_measure)
    if Lost_Step == 0
        delta_d_MPC   = delta_d_measure;
        %delta_d_dot_enhanced = delta_d_dot_measure;
    else
        delta_d_MPC   = delta_d_pre_freeze_if_lost(Lost_Step);
        %delta_d_dot_enhanced = delta_d_dot_pre_freeze_if_lost(Lost_Step); 
    end
end

== matlab function HDVPSG_DelayComp_NewRef_RealDrop_case1/HDV2_control_withPDR_compen/Subsystem1/MATLAB Function3 ==
  data: Lost_Step input; delta_d_pre_freeze_if_lost input; delta_d_measure input; delta_d_MPC output
function delta_d_MPC  = fcn(Lost_Step, delta_d_pre_freeze_if_lost, delta_d_measure)
    if Lost_Step == 0
        delta_d_MPC   = delta_d_measure;
        %delta_d_dot_enhanced = delta_d_dot_measure;
    else
        delta_d_MPC   = delta_d_pre_freeze_if_lost(Lost_Step);
        %delta_d_dot_enhanced = delta_d_dot_pre_freeze_if_lost(Lost_Step); 
    end
end

== matlab function HDVPSG_DelayComp_NewRef_RealDrop_case1/HDV2_control_withPDR_compen/States_update2 ==
  data: x0 output; delta_d input; delta_d_dot input
function x0 = Init(delta_d, delta_d_dot)
    x0 = [delta_d;
          delta_d_dot];
end

== matlab function HDVPSG_DelayComp_NewRef_RealDrop_case1/PSG1_control_withPDR_compen/MATLAB Function ==
  data: REALWORLD_DIST output; X_Ego input; Rho_delta_d_adpt output; Y_Ego input; X_Front input; Y_Front input; DELTA_D_MIN input; Rho_delta_dMAX input
function [REALWORLD_DIST, Rho_delta_d_adpt] = Adaptive_Rho_delta_d(X_Ego, Y_Ego, X_Front, Y_Front, DELTA_D_MIN, Rho_delta_dMAX)
    REALWORLD_DIST = sqrt((X_Ego - X_Front)^2 + (Y_Ego - Y_Front)^2); % The virtual leading car may be in another lane: So far away from the ego_car

    if REALWORLD_DIST>2*DELTA_D_MIN  %  This is determined by the road geometry
        Rho_delta_d_adpt = 0; % Disable 
    elseif REALWORLD_DIST>DELTA_D_MIN
        Rho_delta_d_adpt = -Rho_delta_dMAX/DELTA_D_MIN*REALWORLD_DIST + 2*Rho_delta_dMAX;   % linear adaptive gain
    else
        Rho_delta_d_adpt = Rho_delta_dMAX;
    end
    
end

== matlab function HDVPSG_DelayComp_NewRef_RealDrop_case1/PSG1_control_withPDR_compen/MATLAB Function2 ==
  data: Recv input; Lost_Step output
function Lost_Step = fcn(Recv)
  persistent NUM;
  if isempty(NUM)
      NUM =0;
  end
      
  if Recv == 0
      NUM = NUM +1;
  else
      NUM = 0;
  end
  Lost_Step = NUM;
end

== matlab function HDVPSG_DelayComp_NewRef_RealDrop_case1/PSG1_control_withPDR_compen/Subsystem2/MATLAB Function3 ==
  data: Lost_Step input; delta_d_pre_freeze_if_lost input; delta_d_measure input; delta_d_MPC output
function delta_d_MPC  = fcn(Lost_Step, delta_d_pre_freeze_if_lost, delta_d_measure)
    if Lost_Step == 0
        delta_d_MPC   = delta_d_measure;
        %delta_d_dot_enhanced = delta_d_dot_measure;
    else
        delta_d_MPC   = delta_d_pre_freeze_if_lost(Lost_Step);
        %delta_d_dot_enhanced = delta_d_dot_pre_freeze_if_lost(Lost_Step); 
    end
end

== matlab function HDVPSG_DelayComp_NewRef_RealDrop_case1/ARE_First_Order_Derivative_[1,0,0]11/MATLAB Function ==
  data: U input; Dot_U output; Ts input; u_init input
function Dot_U = buffer(U, Ts, u_init)
    N = 12;
    %Ts = 0.01;
    persistent y;
    if isempty(y)
        y=u_init*ones(N+1,1);%m/s
    end

    y = [U;y(1:end-1)];
    T = Ts*N;
    P = zeros(1,N+1);
    P_alpha = P;
    for k = 1:N+1
        tao_k = (k-1)*Ts;
        P(k) = T-2*tao_k;
        if((k==1)||(k==N+1))
            P_alpha(k) = P(k)*Ts/2;
        else
            P_alpha(k) = P(k)*Ts;
        end
    end
    
    Dot_U = P_alpha*y*6/(T^3);

end

== matlab function HDVPSG_DelayComp_NewRef_RealDrop_case1/ARE_First_Order_Derivative_[1,0,0]12/MATLAB Function ==
  data: U input; Dot_U output; Ts input; u_init input
function Dot_U = buffer(U, Ts, u_init)
    N = 12;
    %Ts = 0.01;
    persistent y;
    if isempty(y)
        y=u_init*ones(N+1,1);%m/s
    end

    y = [U;y(1:end-1)];
    T = Ts*N;
    P = zeros(1,N+1);
    P_alpha = P;
    for k = 1:N+1
        tao_k = (k-1)*Ts;
        P(k) = T-2*tao_k;
        if((k==1)||(k==N+1))
            P_alpha(k) = P(k)*Ts/2;
        else
            P_alpha(k) = P(k)*Ts;
        end
    end
    
    Dot_U = P_alpha*y*6/(T^3);

end

== matlab function HDVPSG_DelayComp_NewRef_RealDrop_case1/ARE_First_Order_Derivative_[1,0,0]13/MATLAB Function ==
  data: U input; Dot_U output; Ts input; u_init input
function Dot_U = buffer(U, Ts, u_init)
    N = 12;
    %Ts = 0.01;
    persistent y;
    if isempty(y)
        y=u_init*ones(N+1,1);%m/s
    end

    y = [U;y(1:end-1)];
    T = Ts*N;
    P = zeros(1,N+1);
    P_alpha = P;
    for k = 1:N+1
        tao_k = (k-1)*Ts;
        P(k) = T-2*tao_k;
        if((k==1)||(k==N+1))
            P_alpha(k) = P(k)*Ts/2;
        else
            P_alpha(k) = P(k)*Ts;
        end
    end
    
    Dot_U = P_alpha*y*6/(T^3);

end

== matlab function HDVPSG_DelayComp_NewRef_RealDrop_case1/ARE_First_Order_Derivative_[1,0,0]14/MATLAB Function ==
  data: U input; Dot_U output; Ts input; u_init input
function Dot_U = buffer(U, Ts, u_init)
    N = 12;
    %Ts = 0.01;
    persistent y;
    if isempty(y)
        y=u_init*ones(N+1,1);%m/s
    end

    y = [U;y(1:end-1)];
    T = Ts*N;
    P = zeros(1,N+1);
    P_alpha = P;
    for k = 1:N+1
        tao_k = (k-1)*Ts;
        P(k) = T-2*tao_k;
        if((k==1)||(k==N+1))
            P_alpha(k) = P(k)*Ts/2;
        else
            P_alpha(k) = P(k)*Ts;
        end
    end
    
    Dot_U = P_alpha*y*6/(T^3);

end

== matlab function HDVPSG_DelayComp_NewRef_RealDrop_case1/ARE_First_Order_Derivative_[1,0,0]15/MATLAB Function ==
  data: U input; Dot_U output; Ts input; u_init input
function Dot_U = buffer(U, Ts, u_init)
    N = 12;
    %Ts = 0.01;
    persistent y;
    if isempty(y)
        y=u_init*ones(N+1,1);%m/s
    end

    y = [U;y(1:end-1)];
    T = Ts*N;
    P = zeros(1,N+1);
    P_alpha = P;
    for k = 1:N+1
        tao_k = (k-1)*Ts;
        P(k) = T-2*tao_k;
        if((k==1)||(k==N+1))
            P_alpha(k) = P(k)*Ts/2;
        else
            P_alpha(k) = P(k)*Ts;
        end
    end
    
    Dot_U = P_alpha*y*6/(T^3);

end

== matlab function HDVPSG_DelayComp_NewRef_RealDrop_case1/Subsystem29/Subsystem7/MATLAB Function ==
  data: distMP input; HighTRFC output
function HighTRFC = fcn(distMP)
    if distMP<=150 && distMP>=120
        HighTRFC = 0; % iced road 
    else 
        HighTRFC = 1;
    end 
end

== matlab function HDVPSG_DelayComp_NewRef_RealDrop_case1/Subsystem2/Subsystem6/MATLAB Function ==
  data: distMP input; HighTRFC output
function HighTRFC = fcn(distMP)
    if distMP<=150 && distMP>=120
        HighTRFC = 0; % iced road 
    else 
        HighTRFC = 1;
    end 
end

== matlab function HDVPSG_DelayComp_NewRef_RealDrop_case1/Subsystem2/Subsystem7/MATLAB Function ==
  data: distMP input; HighTRFC output
function HighTRFC = fcn(distMP)
    if distMP<=150 && distMP>=120
        HighTRFC = 0; % iced road 
    else 
        HighTRFC = 1;
    end 
end

== matlab function HDVPSG_DelayComp_NewRef_RealDrop_case1/Subsystem6/Subsystem7/MATLAB Function ==
  data: distMP input; HighTRFC output
function HighTRFC = fcn(distMP)
    if distMP<=150 && distMP>=120
        HighTRFC = 0; % iced road 
    else 
        HighTRFC = 1;
    end 
end

== matlab function HDVPSG_DelayComp_NewRef_RealDrop_case1/Subsystem3/Subsystem16/MATLAB Function ==
  data: distMP input; HighTRFC output
function HighTRFC = fcn(distMP)
    if distMP<=150 && distMP>=120
        HighTRFC = 0; % iced road 
    else 
        HighTRFC = 1;
    end 
end

== matlab function HDVPSG_DelayComp_NewRef_RealDrop_case1/PSG3_control_withPDR_compen/Sys3 ==
  data: Ts input; A output; B output; dk output; beta input; delta_d_ddot_hat input
function [A, B, dk] = Sys(Ts, beta, delta_d_ddot_hat)
    A = [1  Ts;
         0  1];
    
    B =  [0; -beta*Ts];
    
    dk = [0; delta_d_ddot_hat*Ts];
end

== matlab function HDVPSG_DelayComp_NewRef_RealDrop_case1/HDV2_control_withPDR_compen/PRE_OPT_Pos ==
  data: alpha_pre input; opt_pos_pre output; opt_spd_pre output; beta_pre input; c_1_pre input; c_2_pre input; c_3_pre input; c_4_pre input; v_mp input; T_all_to_MP_pre input; t_aft_trigger_pre input; opt_pos_pre_vec output; opt_spd_pre_vec output
function [opt_pos_pre, opt_spd_pre, opt_pos_pre_vec, opt_spd_pre_vec] = Opt_Pos_Ref_Pre(alpha_pre, beta_pre, c_1_pre, c_2_pre, c_3_pre, c_4_pre, v_mp, T_all_to_MP_pre, t_aft_trigger_pre)
Np              = 20;
opt_pos_pre_vec = zeros(1, Np+1);
opt_spd_pre_vec = zeros(1, Np+1);
%opt_acc_vec = zeros(1, Np+1);

Ts    = 0.01;
 % t = min(t, T_rest_to_MP);
  t_vec = t_aft_trigger_pre + (1:(Np+1))*Ts;
 
 if t_aft_trigger_pre <= T_all_to_MP_pre
     opt_pos_pre = -alpha_pre.*exp(t_aft_trigger_pre) + beta_pre.*exp(-t_aft_trigger_pre) + 1/6.*c_1_pre.*t_aft_trigger_pre.^3 + c_2_pre./2.*t_aft_trigger_pre.^2 + c_3_pre.*t_aft_trigger_pre + c_4_pre;
     opt_spd_pre = -alpha_pre.*exp(t_aft_trigger_pre) - beta_pre.*exp(-t_aft_trigger_pre) + 1/2.*c_1_pre.*t_aft_trigger_pre.^2 + c_2_pre.*t_aft_trigger_pre + c_3_pre;
 else
     opt_pos_pre = v_mp*(t_aft_trigger_pre-T_all_to_MP_pre);
     opt_spd_pre = v_mp;
 end
 
for i = 1:Np+1
    if t_vec(i)<=T_all_to_MP_pre
        opt_pos_pre_vec(i) = -alpha_pre.*exp(t_vec(i)) + beta_pre.*exp(-t_vec(i)) + 1/6.*c_1_pre.*t_vec(i).^3 + c_2_pre./2.*t_vec(i).^2 + c_3_pre.*t_vec(i) + c_4_pre;
        opt_spd_pre_vec(i) = -alpha_pre.*exp(t_vec(i)) - beta_pre.*exp(-t_vec(i)) + 1/2.*c_1_pre.*t_vec(i).^2 + c_2_pre.*t_vec(i)       + c_3_pre;
      %  opt_acc_vec(i) = -alpha.*exp(t_vec(i)) + beta.*exp(-t_vec(i)) + c_1.*t_vec(i) + c_2;
    else
        opt_pos_pre_vec(i) = v_mp*(t_vec(i)-T_all_to_MP_pre); 
        opt_spd_pre_vec(i) = v_mp;
     %   opt_acc_vec(i) = 0; 
    end
end
 
end

== matlab function HDVPSG_DelayComp_NewRef_RealDrop_case1/PSG1_control_withPDR_compen/PRE_OPT_Pos ==
  data: alpha_pre input; opt_pos_pre output; opt_spd_pre output; beta_pre input; c_1_pre input; c_2_pre input; c_3_pre input; c_4_pre input; v_mp input; T_all_to_MP_pre input; t_aft_trigger_pre input; opt_pos_pre_vec output; opt_spd_pre_vec output
function [opt_pos_pre, opt_spd_pre, opt_pos_pre_vec, opt_spd_pre_vec] = Opt_Pos_Ref_Pre(alpha_pre, beta_pre, c_1_pre, c_2_pre, c_3_pre, c_4_pre, v_mp, T_all_to_MP_pre, t_aft_trigger_pre)
Np              = 20;
opt_pos_pre_vec = zeros(1, Np+1);
opt_spd_pre_vec = zeros(1, Np+1);
%opt_acc_vec = zeros(1, Np+1);

Ts    = 0.01;
 % t = min(t, T_rest_to_MP);
  t_vec = t_aft_trigger_pre + (1:(Np+1))*Ts;
 
 if t_aft_trigger_pre <= T_all_to_MP_pre
     opt_pos_pre = -alpha_pre.*exp(t_aft_trigger_pre) + beta_pre.*exp(-t_aft_trigger_pre) + 1/6.*c_1_pre.*t_aft_trigger_pre.^3 + c_2_pre./2.*t_aft_trigger_pre.^2 + c_3_pre.*t_aft_trigger_pre + c_4_pre;
     opt_spd_pre = -alpha_pre.*exp(t_aft_trigger_pre) - beta_pre.*exp(-t_aft_trigger_pre) + 1/2.*c_1_pre.*t_aft_trigger_pre.^2 + c_2_pre.*t_aft_trigger_pre + c_3_pre;
 else
     opt_pos_pre = v_mp*(t_aft_trigger_pre-T_all_to_MP_pre);
     opt_spd_pre = v_mp;
 end
 
for i = 1:Np+1
    if t_vec(i)<=T_all_to_MP_pre
        opt_pos_pre_vec(i) = -alpha_pre.*exp(t_vec(i)) + beta_pre.*exp(-t_vec(i)) + 1/6.*c_1_pre.*t_vec(i).^3 + c_2_pre./2.*t_vec(i).^2 + c_3_pre.*t_vec(i) + c_4_pre;
        opt_spd_pre_vec(i) = -alpha_pre.*exp(t_vec(i)) - beta_pre.*exp(-t_vec(i)) + 1/2.*c_1_pre.*t_vec(i).^2 + c_2_pre.*t_vec(i)       + c_3_pre;
      %  opt_acc_vec(i) = -alpha.*exp(t_vec(i)) + beta.*exp(-t_vec(i)) + c_1.*t_vec(i) + c_2;
    else
        opt_pos_pre_vec(i) = v_mp*(t_vec(i)-T_all_to_MP_pre); 
        opt_spd_pre_vec(i) = v_mp;
     %   opt_acc_vec(i) = 0; 
    end
end
 
end

== matlab function HDVPSG_DelayComp_NewRef_RealDrop_case1/PSG1_control_withPDR_compen/SELF_Optimal_Control_Reference ==
  data: opt_spd output; L_ctz input; opt_pos output; v_ini input; a_ini input; T_all_to_MP input; v_mp input; t_aft_trigger input; opt_acc output; opt_pos_vec output; opt_spd_vec output; alpha output; beta output; c_1 output; c_2 output; c_3 output; c_4 output
function [opt_spd, opt_pos, opt_acc, opt_pos_vec, opt_spd_vec, alpha, beta, c_1, c_2, c_3, c_4] = Opt_Ref(L_ctz, v_ini, a_ini, T_all_to_MP, v_mp, t_aft_trigger)
Np          = 20;
opt_pos_vec = zeros(1, Np+1);
opt_spd_vec = zeros(1, Np+1);
%opt_acc_vec = zeros(1, Np+1);

Ts    = 0.01;
L_ctz = -L_ctz;

alpha = -(12*v_mp - 12*v_ini - 12*L_ctz - 6*T_all_to_MP*a_ini - 12*T_all_to_MP*v_mp + 6*T_all_to_MP*L_ctz + 2*T_all_to_MP^2*a_ini + 2*T_all_to_MP^2*v_ini + 4*T_all_to_MP^2*v_mp + 12*v_ini*exp(-T_all_to_MP) - 12*v_mp*exp(-T_all_to_MP) + 12*L_ctz*exp(-T_all_to_MP) + 6*T_all_to_MP*a_ini*exp(-T_all_to_MP) + 12*T_all_to_MP*v_ini*exp(-T_all_to_MP) + 6*T_all_to_MP*L_ctz*exp(-T_all_to_MP) + 4*T_all_to_MP^2*a_ini*exp(-T_all_to_MP) + T_all_to_MP^3*a_ini*exp(-T_all_to_MP) + 4*T_all_to_MP^2*v_ini*exp(-T_all_to_MP) + 2*T_all_to_MP^2*v_mp*exp(-T_all_to_MP))/(24*exp(-T_all_to_MP) + 24*exp(T_all_to_MP) + 8*T_all_to_MP^2*exp(-T_all_to_MP) + T_all_to_MP^3*exp(-T_all_to_MP) - 24*T_all_to_MP*exp(T_all_to_MP) + 8*T_all_to_MP^2 + 24*T_all_to_MP*exp(-T_all_to_MP) + 8*T_all_to_MP^2*exp(T_all_to_MP) - T_all_to_MP^3*exp(T_all_to_MP) - 48);

beta  = -(12*v_mp - 12*v_ini + 12*L_ctz - 6*T_all_to_MP*a_ini + 12*T_all_to_MP*v_mp + 6*T_all_to_MP*L_ctz - 2*T_all_to_MP^2*a_ini + 2*T_all_to_MP^2*v_ini + 4*T_all_to_MP^2*v_mp + 12*v_ini*exp(T_all_to_MP) - 12*v_mp*exp(T_all_to_MP) - 12*L_ctz*exp(T_all_to_MP) - 4*T_all_to_MP^2*a_ini*exp(T_all_to_MP) + T_all_to_MP^3*a_ini*exp(T_all_to_MP) + 4*T_all_to_MP^2*v_ini*exp(T_all_to_MP) + 2*T_all_to_MP^2*v_mp*exp(T_all_to_MP) + 6*T_all_to_MP*a_ini*exp(T_all_to_MP) - 12*T_all_to_MP*v_ini*exp(T_all_to_MP) + 6*T_all_to_MP*L_ctz*exp(T_all_to_MP))/(24*exp(-T_all_to_MP) + 24*exp(T_all_to_MP) + 8*T_all_to_MP^2*exp(-T_all_to_MP) + T_all_to_MP^3*exp(-T_all_to_MP) - 24*T_all_to_MP*exp(T_all_to_MP) + 8*T_all_to_MP^2 + 24*T_all_to_MP*exp(-T_all_to_MP) + 8*T_all_to_MP^2*exp(T_all_to_MP) - T_all_to_MP^3*exp(T_all_to_MP) - 48);

  c_1 = -(6*(8*L_ctz - 8*a_ini + 4*T_all_to_MP*v_ini + 4*T_all_to_MP*v_mp + 2*T_all_to_MP^2*a_ini + 4*a_ini*exp(T_all_to_MP) - 4*L_ctz*exp(T_all_to_MP) + 4*a_ini*exp(-T_all_to_MP) - 4*L_ctz*exp(-T_all_to_MP) + 4*T_all_to_MP*a_ini*exp(-T_all_to_MP) + T_all_to_MP^2*a_ini*exp(T_all_to_MP) - 2*T_all_to_MP*v_ini*exp(-T_all_to_MP) + T_all_to_MP^2*v_ini*exp(T_all_to_MP) - 2*T_all_to_MP*v_mp*exp(-T_all_to_MP) + T_all_to_MP^2*v_mp*exp(T_all_to_MP) - 2*T_all_to_MP*L_ctz*exp(-T_all_to_MP) + T_all_to_MP^2*a_ini*exp(-T_all_to_MP) - T_all_to_MP^2*v_ini*exp(-T_all_to_MP) - T_all_to_MP^2*v_mp*exp(-T_all_to_MP) - 4*T_all_to_MP*a_ini*exp(T_all_to_MP) - 2*T_all_to_MP*v_ini*exp(T_all_to_MP) - 2*T_all_to_MP*v_mp*exp(T_all_to_MP) + 2*T_all_to_MP*L_ctz*exp(T_all_to_MP)))/(T_all_to_MP*(24*exp(-T_all_to_MP) + 24*exp(T_all_to_MP) + 8*T_all_to_MP^2*exp(-T_all_to_MP) + T_all_to_MP^3*exp(-T_all_to_MP) - 24*T_all_to_MP*exp(T_all_to_MP) + 8*T_all_to_MP^2 + 24*T_all_to_MP*exp(-T_all_to_MP) + 8*T_all_to_MP^2*exp(T_all_to_MP) - T_all_to_MP^3*exp(T_all_to_MP) - 48)); 
  
  c_2 = (2*(12*L_ctz - 24*a_ini + 12*T_all_to_MP*v_mp + 2*T_all_to_MP^2*a_ini + 12*a_ini*exp(T_all_to_MP) + 6*v_ini*exp(T_all_to_MP) - 6*v_mp*exp(T_all_to_MP) - 6*L_ctz*exp(T_all_to_MP) + 12*a_ini*exp(-T_all_to_MP) - 6*v_ini*exp(-T_all_to_MP) + 6*v_mp*exp(-T_all_to_MP) - 6*L_ctz*exp(-T_all_to_MP) + 9*T_all_to_MP*a_ini*exp(-T_all_to_MP) + 2*T_all_to_MP^2*a_ini*exp(T_all_to_MP) - 6*T_all_to_MP*v_ini*exp(-T_all_to_MP) + 2*T_all_to_MP^2*v_ini*exp(T_all_to_MP) + T_all_to_MP^2*v_mp*exp(T_all_to_MP) - 3*T_all_to_MP*L_ctz*exp(-T_all_to_MP) + 2*T_all_to_MP^2*a_ini*exp(-T_all_to_MP) - 2*T_all_to_MP^2*v_ini*exp(-T_all_to_MP) - T_all_to_MP^2*v_mp*exp(-T_all_to_MP) - 9*T_all_to_MP*a_ini*exp(T_all_to_MP) - 6*T_all_to_MP*v_ini*exp(T_all_to_MP) + 3*T_all_to_MP*L_ctz*exp(T_all_to_MP)))/(24*exp(-T_all_to_MP) + 24*exp(T_all_to_MP) + 8*T_all_to_MP^2*exp(-T_all_to_MP) + T_all_to_MP^3*exp(-T_all_to_MP) - 24*T_all_to_MP*exp(T_all_to_MP) + 8*T_all_to_MP^2 + 24*T_all_to_MP*exp(-T_all_to_MP) + 8*T_all_to_MP^2*exp(T_all_to_MP) - T_all_to_MP^3*exp(T_all_to_MP) - 48); 
  
  c_3 = -(24*v_ini + 24*v_mp - 12*T_all_to_MP*a_ini + 12*T_all_to_MP*L_ctz - 4*T_all_to_MP^2*v_ini + 8*T_all_to_MP^2*v_mp - 12*v_ini*exp(T_all_to_MP) - 12*v_mp*exp(T_all_to_MP) - 12*L_ctz*exp(T_all_to_MP) - 12*v_ini*exp(-T_all_to_MP) - 12*v_mp*exp(-T_all_to_MP) + 12*L_ctz*exp(-T_all_to_MP) + 6*T_all_to_MP*a_ini*exp(-T_all_to_MP) - 4*T_all_to_MP^2*a_ini*exp(T_all_to_MP) + T_all_to_MP^3*a_ini*exp(T_all_to_MP) - 12*T_all_to_MP*v_ini*exp(-T_all_to_MP) - 4*T_all_to_MP^2*v_ini*exp(T_all_to_MP) + T_all_to_MP^3*v_ini*exp(T_all_to_MP) + 2*T_all_to_MP^2*v_mp*exp(T_all_to_MP) + 6*T_all_to_MP*L_ctz*exp(-T_all_to_MP) + 4*T_all_to_MP^2*a_ini*exp(-T_all_to_MP) + T_all_to_MP^3*a_ini*exp(-T_all_to_MP) - 4*T_all_to_MP^2*v_ini*exp(-T_all_to_MP) - T_all_to_MP^3*v_ini*exp(-T_all_to_MP) + 2*T_all_to_MP^2*v_mp*exp(-T_all_to_MP) + 6*T_all_to_MP*a_ini*exp(T_all_to_MP) + 12*T_all_to_MP*v_ini*exp(T_all_to_MP) + 6*T_all_to_MP*L_ctz*exp(T_all_to_MP))/(24*exp(-T_all_to_MP) + 24*exp(T_all_to_MP) + 8*T_all_to_MP^2*exp(-T_all_to_MP) + T_all_to_MP^3*exp(-T_all_to_MP) - 24*T_all_to_MP*exp(T_all_to_MP) + 8*T_all_to_MP^2 + 24*T_all_to_MP*exp(-T_all_to_MP) + 8*T_all_to_MP^2*exp(T_all_to_MP) - T_all_to_MP^3*exp(T_all_to_MP) - 48); 
  
  c_4 = -(24*L_ctz - 24*T_all_to_MP*v_mp + 4*T_all_to_MP^2*a_ini - 8*T_all_to_MP^2*L_ctz - 12*v_ini*exp(T_all_to_MP) + 12*v_mp*exp(T_all_to_MP) - 12*L_ctz*exp(T_all_to_MP) + 12*v_ini*exp(-T_all_to_MP) - 12*v_mp*exp(-T_all_to_MP) - 12*L_ctz*exp(-T_all_to_MP) + 6*T_all_to_MP*a_ini*exp(-T_all_to_MP) + 4*T_all_to_MP^2*a_ini*exp(T_all_to_MP) - T_all_to_MP^3*a_ini*exp(T_all_to_MP) + 12*T_all_to_MP*v_ini*exp(-T_all_to_MP) - 4*T_all_to_MP^2*v_ini*exp(T_all_to_MP) - 2*T_all_to_MP^2*v_mp*exp(T_all_to_MP) - 18*T_all_to_MP*L_ctz*exp(-T_all_to_MP) - 8*T_all_to_MP^2*L_ctz*exp(T_all_to_MP) + T_all_to_MP^3*L_ctz*exp(T_all_to_MP) + 4*T_all_to_MP^2*a_ini*exp(-T_all_to_MP) + T_all_to_MP^3*a_ini*exp(-T_all_to_MP) + 4*T_all_to_MP^2*v_ini*exp(-T_all_to_MP) + 2*T_all_to_MP^2*v_mp*exp(-T_all_to_MP) - 8*T_all_to_MP^2*L_ctz*exp(-T_all_to_MP) - T_all_to_MP^3*L_ctz*exp(-T_all_to_MP) - 6*T_all_to_MP*a_ini*exp(T_all_to_MP) + 12*T_all_to_MP*v_ini*exp(T_all_to_MP) + 18*T_all_to_MP*L_ctz*exp(T_all_to_MP))/(24*exp(-T_all_to_MP) + 24*exp(T_all_to_MP) + 8*T_all_to_MP^2*exp(-T_all_to_MP) + T_all_to_MP^3*exp(-T_all_to_MP) - 24*T_all_to_MP*exp(T_all_to_MP) + 8*T_all_to_MP^2 + 24*T_all_to_MP*exp(-T_all_to_MP) + 8*T_all_to_MP^2*exp(T_all_to_MP) - T_all_to_MP^3*exp(T_all_to_MP) - 48);
  
 % t = min(t, T_rest_to_MP);
  t_vec = t_aft_trigger + (1:(Np+1))*Ts;
 
 if t_aft_trigger <= T_all_to_MP
     opt_pos = -alpha.*exp(t_aft_trigger) + beta.*exp(-t_aft_trigger) + 1/6.*c_1.*t_aft_trigger.^3 + c_2./2.*t_aft_trigger.^2 + c_3.*t_aft_trigger + c_4;
     opt_spd = -alpha.*exp(t_aft_trigger) - beta.*exp(-t_aft_trigger) + 1/2.*c_1.*t_aft_trigger.^2 + c_2.*t_aft_trigger + c_3;
     opt_acc = -alpha.*exp(t_aft_trigger) + beta.*exp(-t_aft_trigger) + c_1.*t_aft_trigger + c_2;
 else
     opt_pos = v_mp*(t_aft_trigger-T_all_to_MP);
     opt_spd = v_mp;
     opt_acc = 0;
 end
 
for i = 1:Np+1
    if t_vec(i)<=T_all_to_MP
        opt_pos_vec(i) = -alpha.*exp(t_vec(i)) + beta.*exp(-t_vec(i)) + 1/6.*c_1.*t_vec(i).^3 + c_2./2.*t_vec(i).^2 + c_3.*t_vec(i) + c_4;
        opt_spd_vec(i) = -alpha.*exp(t_vec(i)) - beta.*exp(-t_vec(i)) + 1/2.*c_1.*t_vec(i).^2 + c_2.*t_vec(i)       + c_3;
      %  opt_acc_vec(i) = -alpha.*exp(t_vec(i)) + beta.*exp(-t_vec(i)) + c_1.*t_vec(i) + c_2;
    else
        opt_pos_vec(i) = v_mp*(t_vec(i)-T_all_to_MP); 
        opt_spd_vec(i) = v_mp;
     %   opt_acc_vec(i) = 0; 
    end
end
 
end

== matlab function HDVPSG_DelayComp_NewRef_RealDrop_case1/PSG1_control_withPDR_compen/States_update2 ==
  data: x0 output; delta_d input; delta_d_dot input
function x0 = Init(delta_d, delta_d_dot)
    x0 = [delta_d;
          delta_d_dot];
end

== matlab function HDVPSG_DelayComp_NewRef_RealDrop_case1/PSG1_control_withPDR_compen/Subsystem17/Poly_coefficient ==
  data: a_0 output; delta_d0 input; a_1 output; a_2 output; delta_dTCC input; delta_v0 input; Tend input; a_3 output
function [a_0, a_1, a_2, a_3] = poly_4_coefficient(delta_d0, delta_dTCC, delta_v0, Tend)
% With conditions:
% delta_d_0 given,            delta_v_0 given 
% delta_d_Tend = delta_d_TTC, delta_v_Tend = 0

% delta_dr(t) = a0 + a1*t + a2*t^2 + a3*t^3
    a_0 = delta_d0;
    a_1 = delta_v0;
    a_2 = -(3*delta_d0 - 3*delta_dTCC + 2*Tend*delta_v0)/Tend^2;
    a_3 = (2*delta_d0 - 2*delta_dTCC + Tend*delta_v0)/Tend^3;
end

== matlab function HDVPSG_DelayComp_NewRef_RealDrop_case1/PSG1_control_withPDR_compen/Subsystem18/Ref ==
  data: delta_dr output; a_0 input; delta_dr_dot output; a_1 input; a_2 input; a_3 input; t_sumo input
function [delta_dr, delta_dr_dot] = poly_4_reference(a_0, a_1, a_2, a_3, t_sumo)
    delta_dr     = a_0 + a_1*t_sumo + a_2*t_sumo^2 + a_3*t_sumo^3;
    delta_dr_dot =       a_1        + 2*a_2*t_sumo + 3*a_3*t_sumo^2;
end

== matlab function HDVPSG_DelayComp_NewRef_RealDrop_case1/PSG1_control_withPDR_compen/Subsystem18/Ref_Pre_Vec ==
  data: delta_dr_Pre_Vec output; a_0 input; delta_dr_dot_Pre_Vec output; a_1 input; a_2 input; a_3 input; t_sumo input
function [delta_dr_Pre_Vec, delta_dr_dot_Pre_Vec] = poly_4_reference(a_0, a_1, a_2, a_3, t_sumo)
    Ts = 0.01;
    Np = 20;
    
    t_Pre_Vec = t_sumo + (1:Np+1)*Ts;
    
    delta_dr_Pre_Vec     = a_0 + a_1*t_Pre_Vec + a_2*t_Pre_Vec.^2 + a_3*t_Pre_Vec.^3;
    delta_dr_dot_Pre_Vec =       a_1           + 2*a_2*t_Pre_Vec  + 3*a_3*t_Pre_Vec.^2;
end

== matlab function HDVPSG_DelayComp_NewRef_RealDrop_case1/Subsystem6/Subsystem18/MATLAB Function ==
  data: distMP input; HighTRFC output
function HighTRFC = fcn(distMP)
    if distMP<=150 && distMP>=120
        HighTRFC = 0; % iced road 
    else 
        HighTRFC = 1;
    end 
end
